simulink model "part1_Simulation4"  (R2014b)
settings: Solver=VariableStepAuto  StartTime=0.0  StopTime=10  RelTol=1e-3
values from neighbouring files (symbols this model uses):
  getPos = [0; 0; 1]    [init_Sim1.m]    (also in init_Sim3.m; init_Sim4.m)
  getVel = [0;1;0]    [init_Sim1.m]    (also in init_Sim3.m; init_Sim4.m)
  Kd = 7*[M3(1)*Omega 0 0; 0 M3(2,2)*Omega 0; 0 0 20*M(3,3)*Omega]    [init_Sim1.m]    (also in init_Sim3.m; init_Sim4.m)
  Ki = 100*(omega/10)*[M3(1)*omega^2 0 0;0 M3(2,2)*omega^2 0; 0 0 M3(3,3)*omega^2 ]*2    [init_Sim1.m]    (also in init_Sim3.m; init_Sim4.m)
  Kp = 50*[M3(1)*omega^2 0 0;0 M3(2,2)*omega^2 0; 0 0 15*M3(3,3)*omega^2 ]    [init_Sim1.m]    (also in init_Sim3.m; init_Sim4.m)
  Omega = 2*damping*omega    [init_Sim1.m]    (also in init_Sim3.m; init_Sim4.m)
  omega = omegab/sqrt(1-2*damping^2+sqrt(4*damping^4-4*damping^2+2))    [init_Sim1.m]    (also in init_Sim3.m; init_Sim4.m)
  ref = [50;0;0]    [init_Sim1.m]    (also in init_Sim3.m = [10 10 -pi/2]; init_Sim4.m = [0;0;0])
  ref1 = [50;0;0]    [init_Sim4.m]
  ref2 = [50;-50;0]    [init_Sim4.m]
  ref3 = [0 -50 -pi/2]    [init_Sim4.m]
  ref4 = [0 0 -pi/2]    [init_Sim4.m]
undefined symbols (not defined in the file or in its folder): Hoerner, vessel
libraries: marine_hydro x1
settings Model: Creator=jonbjor  LastModifiedBy=Karianne
settings DataIOCC: LimitDataPoints=off  SaveFormat=Dataset
settings OptimizationCC: UseDivisionForNetSlopeComputation=off  LifeSpan=auto  SimCompilerOptimization=off
settings DebuggingCC: SolverPrmCheckMsg=none  FcnCallInpInsideContextMsg=error  FrameProcessingCompatibilityMsg=error  SFUnexpectedBacktrackingDiag=error  SFNoUnconditionalDefaultTransitionDiag=error
settings HardwareCC: ProdBitPerPointer=64  ProdLargestAtomicFloat=Float  ProdIntDivRoundTo=Zero  ProdEndianess=LittleEndian  ProdWordSize=64  ProdHWDeviceType=Intel->x86-64 (Windows64)
settings ModelReferenceCC: PropagateSignalLabelsOutOfModel=on
settings RTWCC: RTWCompilerOptimization=off
settings GRTTargetCC: TargetLangStandard=C99 (ISO)  GeneratePreprocessorConditionals=Use local settings

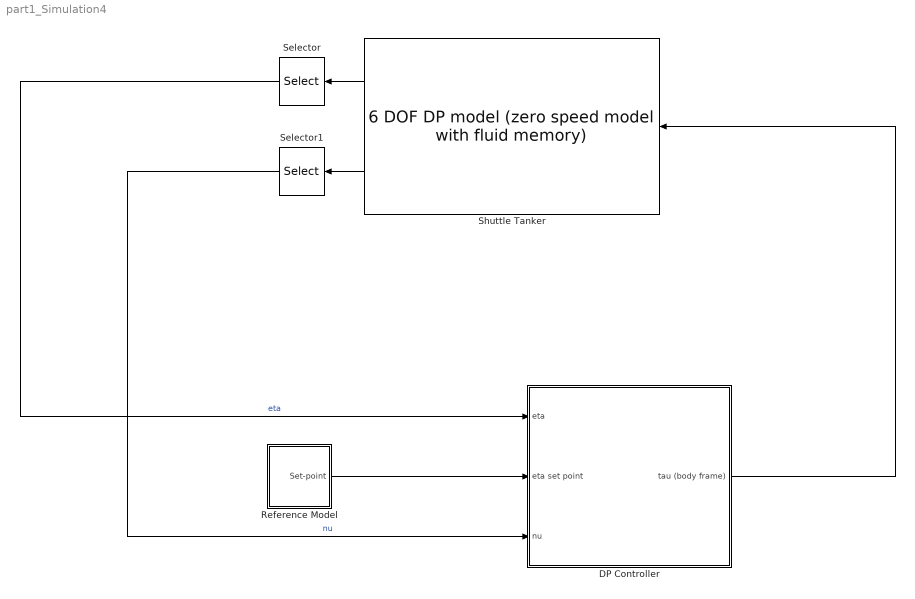
== system part1_Simulation4 ==
  DP Controller : Subsystem
  Reference Model : Subsystem
  Selector : Selector  InputPortWidth=6  Indices=[1 2 6]
  Selector1 : Selector  InputPortWidth=6  Indices=[1 2 6]
  Shuttle Tanker : marine_hydro/Hydro Library/6 DOF DP model  (zero speed model with fluid memory)  ABC=vesselABC  rho=1025  Axc=0.9*vessel.main.T*vessel.main.B  Ayc=0.9*vessel.main.T*vessel.main.Lpp  CX=1  CY_2D=Hoerner(vessel.main.B,vessel.main.T)  Bv=vessel.Bv
      link override "Integrator1 ": InitialCondition=nu0
      link override Integrator2: InitialCondition=eta0
  wires:
  DP Controller/1(tau (body frame)) -> Shuttle Tanker/2
  Shuttle Tanker/1 -> Selector/1
  Shuttle Tanker/2 -> Selector1/1
  Reference Model/1(Set-point) -> DP Controller/2(eta set point)
  Selector1/1 -> DP Controller/3(nu)  "nu"
  Selector/1 -> DP Controller/1(eta)  "eta"

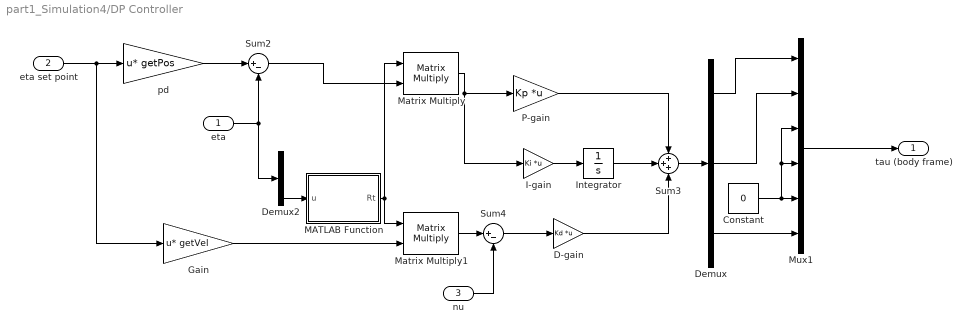
== system part1_Simulation4/DP Controller ==
  eta : Inport
  eta set point : Inport  Port=2
  nu : Inport  Port=3
  Constant : Constant  Value=0
  D-gain : Gain  Gain=Kd  Multiplication=Matrix(K*u)  SaturateOnIntegerOverflow=off  OutDataTypeStr=Inherit: Inherit via internal rule  ParamDataTypeStr=Inherit: Inherit via internal rule
  Demux : Demux  Outputs=3
  Demux2 : Demux  Outputs=3
  Gain : Gain  Gain=getVel  Multiplication=Matrix(u*K)  SaturateOnIntegerOverflow=off  OutDataTypeStr=Inherit: Inherit via internal rule  ParamDataTypeStr=Inherit: Inherit via internal rule
  I-gain : Gain  Gain=Ki  Multiplication=Matrix(K*u)  SaturateOnIntegerOverflow=off  OutDataTypeStr=Inherit: Inherit via internal rule  ParamDataTypeStr=Inherit: Inherit via internal rule
  Integrator : Integrator
  MATLAB Function : MATLAB Function  TreatAsAtomicUnit=on
  Matrix Multiply : Product  Multiplication=Matrix(*)  SaturateOnIntegerOverflow=off  RndMeth=Floor  InputSameDT=off  OutDataTypeStr=Inherit: Inherit via internal rule
  Matrix Multiply1 : Product  Multiplication=Matrix(*)  SaturateOnIntegerOverflow=off  RndMeth=Floor  InputSameDT=off  OutDataTypeStr=Inherit: Inherit via internal rule
  Mux1 : Mux  Inputs=6
  P-gain : Gain  Gain=Kp  Multiplication=Matrix(K*u)  SaturateOnIntegerOverflow=off  OutDataTypeStr=Inherit: Inherit via internal rule  ParamDataTypeStr=Inherit: Inherit via internal rule
  Sum2 : Sum  Inputs=|+-  SaturateOnIntegerOverflow=off  InputSameDT=off  OutDataTypeStr=Inherit: Inherit via internal rule
  Sum3 : Sum  Inputs=+++  SaturateOnIntegerOverflow=off  InputSameDT=off  OutDataTypeStr=Inherit: Inherit via internal rule
  Sum4 : Sum  Inputs=|+-  SaturateOnIntegerOverflow=off  InputSameDT=off  OutDataTypeStr=Inherit: Inherit via internal rule
  pd : Gain  Gain=getPos  Multiplication=Matrix(u*K)  SaturateOnIntegerOverflow=off  OutDataTypeStr=Inherit: Inherit via internal rule  ParamDataTypeStr=Inherit: Inherit via internal rule
  tau (body frame) : Outport
  wires:
  eta set point/1 -> Gain/1, pd/1
  eta/1 -> Sum2/2, Demux2/1
  I-gain/1 -> Integrator/1
  Sum3/1 -> Demux/1
  Demux/1 -> Mux1/1
  Demux/2 -> Mux1/2
  Demux/3 -> Mux1/6
  Constant/1 -> Mux1/4, Mux1/3, Mux1/5
  Mux1/1 -> tau (body frame)/1
  Demux2/3 -> MATLAB Function/1(u)
  nu/1 -> Sum4/2
  Matrix Multiply1/1 -> Sum4/1
  Sum4/1 -> D-gain/1
  P-gain/1 -> Sum3/1
  Matrix Multiply/1 -> I-gain/1, P-gain/1
  Integrator/1 -> Sum3/2
  D-gain/1 -> Sum3/3
  Sum2/1 -> Matrix Multiply/2
  MATLAB Function/1(Rt) -> Matrix Multiply/1, Matrix Multiply1/1
  pd/1 -> Sum2/1
  Gain/1 -> Matrix Multiply1/2

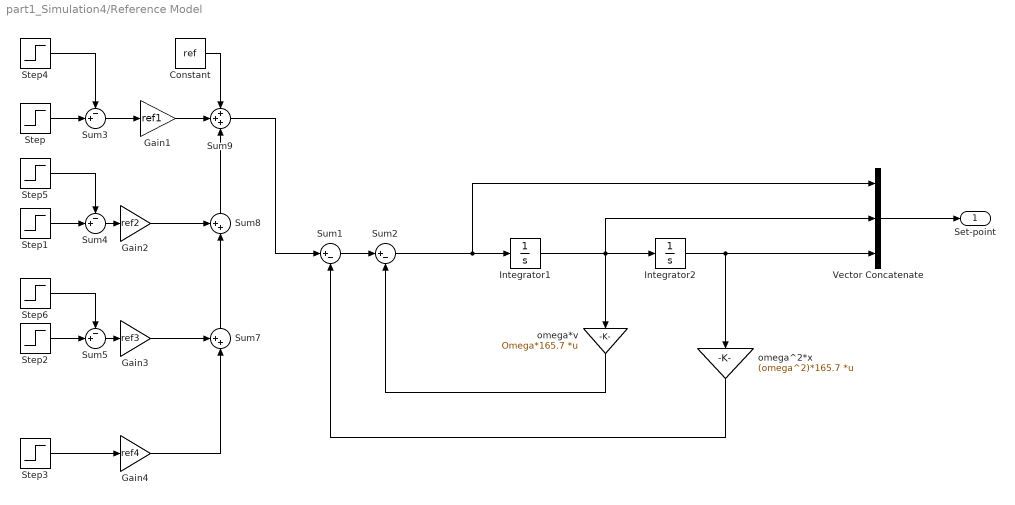
== system part1_Simulation4/Reference Model ==
  Constant : Constant  Value=ref
  Gain1 : Gain  Gain=ref1  SaturateOnIntegerOverflow=off  OutDataTypeStr=Inherit: Inherit via internal rule  ParamDataTypeStr=Inherit: Inherit via internal rule
  Gain2 : Gain  Gain=ref2  SaturateOnIntegerOverflow=off  OutDataTypeStr=Inherit: Inherit via internal rule  ParamDataTypeStr=Inherit: Inherit via internal rule
  Gain3 : Gain  Gain=ref3  SaturateOnIntegerOverflow=off  OutDataTypeStr=Inherit: Inherit via internal rule  ParamDataTypeStr=Inherit: Inherit via internal rule
  Gain4 : Gain  Gain=ref4  SaturateOnIntegerOverflow=off  OutDataTypeStr=Inherit: Inherit via internal rule  ParamDataTypeStr=Inherit: Inherit via internal rule
  Integrator1 : Integrator
  Integrator2 : Integrator
  Step : Step  Time=50  SampleTime=0
  Step1 : Step  Time=200  SampleTime=0
  Step2 : Step  Time=350  SampleTime=0
  Step3 : Step  Time=500  SampleTime=0
  Step4 : Step  Time=200  SampleTime=0
  Step5 : Step  Time=350  SampleTime=0
  Step6 : Step  Time=500  SampleTime=0
  Sum1 : Sum  Inputs=|+-  SaturateOnIntegerOverflow=off  InputSameDT=off  OutDataTypeStr=Inherit: Inherit via internal rule
  Sum2 : Sum  Inputs=|+-  SaturateOnIntegerOverflow=off  InputSameDT=off  OutDataTypeStr=Inherit: Inherit via internal rule
  Sum3 : Sum  Inputs=-+|  SaturateOnIntegerOverflow=off  InputSameDT=off  OutDataTypeStr=Inherit: Inherit via internal rule
  Sum4 : Sum  Inputs=-+|  SaturateOnIntegerOverflow=off  InputSameDT=off  OutDataTypeStr=Inherit: Inherit via internal rule
  Sum5 : Sum  Inputs=-+|  SaturateOnIntegerOverflow=off  InputSameDT=off  OutDataTypeStr=Inherit: Inherit via internal rule
  Sum7 : Sum  Inputs=++|  SaturateOnIntegerOverflow=off  InputSameDT=off  OutDataTypeStr=Inherit: Inherit via internal rule
  Sum8 : Sum  Inputs=++|  SaturateOnIntegerOverflow=off  InputSameDT=off  OutDataTypeStr=Inherit: Inherit via internal rule
  Sum9 : Sum  Inputs=+++  SaturateOnIntegerOverflow=off  InputSameDT=off  OutDataTypeStr=Inherit: Inherit via internal rule
  Vector Concatenate : Concatenate  NumInputs=3  Mode=Multidimensional array  ConcatenateDimension=2
  omega*v : Gain  Gain=Omega*165.7  Multiplication=Matrix(K*u)  SaturateOnIntegerOverflow=off  OutDataTypeStr=Inherit: Inherit via internal rule  ParamDataTypeStr=Inherit: Inherit via internal rule
  omega^2*x : Gain  Gain=(omega^2)*165.7  Multiplication=Matrix(K*u)  SaturateOnIntegerOverflow=off  OutDataTypeStr=Inherit: Inherit via internal rule  ParamDataTypeStr=Inherit: Inherit via internal rule
  Set-point : Outport
  wires:
  omega^2*x/1 -> Sum1/2
  Vector Concatenate/1 -> Set-point/1
  Sum1/1 -> Sum2/1
  omega*v/1 -> Sum2/2
  Integrator2/1 -> Vector Concatenate/3, omega^2*x/1
  Integrator1/1 -> Vector Concatenate/2, omega*v/1, Integrator2/1
  Sum2/1 -> Vector Concatenate/1, Integrator1/1
  Sum3/1 -> Gain1/1
  Step/1 -> Sum3/2
  Step4/1 -> Sum3/1
  Step1/1 -> Sum4/2
  Step5/1 -> Sum4/1
  Sum4/1 -> Gain2/1
  Step2/1 -> Sum5/2
  Step6/1 -> Sum5/1
  Sum5/1 -> Gain3/1
  Step3/1 -> Gain4/1
  Gain4/1 -> Sum7/2
  Gain3/1 -> Sum7/1
  Sum7/1 -> Sum8/2
  Gain2/1 -> Sum8/1
  Sum9/1 -> Sum1/1
  Sum8/1 -> Sum9/3
  Gain1/1 -> Sum9/2
  Constant/1 -> Sum9/1

== matlab function part1_Simulation4/DP Controller/MATLAB Function ==
  data: u input; Rt output
function Rt = fcn(u)

R=[cos(u) -sin(u) 0; sin(u) cos(u) 0; 0 0 1];
Rt=transpose(R);

end
